simulink subsystem "s0307_theta_controller_PID"  (R2019b)
settings: Solver=VariableStepAuto  StartTime=0.0  StopTime=10.0  RelTol=1e-3
model mask{wc=0, cz_ratio=0, pc_ratio=0}
  mask prompts: wc "Cutting Frequency"; cz_ratio "Cutting/Zeros Frequency Ratio"; pc_ratio "Pole/Cutting Frequency Ratio"
undefined symbols (not defined in the file): dt_control, PARAMS
libraries: simulink x1
settings Model: Creator=paolo  LastModifiedBy=paolo
settings DebuggingCC: SFMachineParentedDataDiag=error

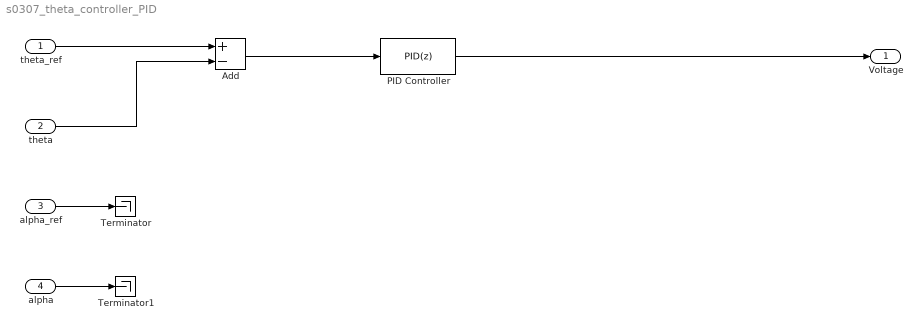
== system s0307_theta_controller_PID ==
  theta_ref : Inport
  theta : Inport  Port=2
  alpha_ref : Inport  Port=3
  alpha : Inport  Port=4
  Add : Sum  Inputs=+-
  PID Controller : simulink/Continuous/PID Controller  Controller=PID  Form=Parallel  TimeDomain=Discrete-time  SampleTime=dt_control  IntegratorMethod=Trapezoidal  FilterMethod=Trapezoidal  ControllerParametersSource=internal  P=wc^2 * (2 * cz_ratio * pc_ratio - 1) / (cz_ratio^2 * pc_ratio * PARAMS.mu_V_theta_dot)  I=wc^3 / PARAMS.mu_V_theta_dot / cz_ratio^2  D="wc * (cz_ratio^2 * pc_ratio^2 - 2 * cz_ratio * pc_ratio + 1)  / (cz_ratio^2 * pc_ratio^2 * PARAMS.mu_V_theta_dot)"  UseFilter=on  N=pc_ratio * wc  TunerSelectOption=Frequency Response Based  InitialConditionSource=internal  InitialConditionForIntegrator=0  InitialConditionForFilter=0  DifferentiatorICPrevScaledInput=0  ExternalReset=none  TrackingMode=off  Kt=1  LimitOutput=on  UpperSaturationLimit=PARAMS.V_sat  LowerSaturationLimit=-PARAMS.V_sat  LinearizeAsGain=on  AntiWindupMode=clamping  Kb=1  POutMin=[]  POutMax=[]  IOutMin=[]  IOutMax=[]  DOutMin=[]  DOutMax=[]  NOutMin=[]  NOutMax=[]  SumOutMin=[]  SumOutMax=[]  SaturationOutMin=[]  SaturationOutMax=[]  PParamMin=[]  PParamMax=[]  IParamMin=[]  IParamMax=[]  DParamMin=[]  DParamMax=[]  NParamMin=[]  NParamMax=[]  KbParamMin=[]  KbParamMax=[]  KtParamMin=[]  KtParamMax=[]  KbOutMin=[]  KbOutMax=[]  KtOutMin=[]  KtOutMax=[]  IntegratorOutMin=[]  IntegratorOutMax=[]  FilterOutMin=[]  FilterOutMax=[]  SumI1OutMin=[]  SumI1OutMax=[]  SumI2OutMin=[]  SumI2OutMax=[]  SumI3OutMin=[]  SumI3OutMax=[]  SumI4OutMin=[]  SumI4OutMax=[]  SumDOutMin=[]  SumDOutMax=[]  DifferentiatorOutMin=[]  DifferentiatorOutMax=[]  FilterDiffOutCoefMin=[]  FilterDiffOutCoefMax=[]  ReciprocalOutMin=[]  ReciprocalOutMax=[]  SumDenOutMin=[]  SumDenOutMax=[]  SumNumOutMin=[]  SumNumOutMax=[]  DivideOutMin=[]  DivideOutMax=[]  IntegratorContinuousStateAttributes=''  IntegratorStateMustResolveToSignalObject=off  IntegratorRTWStateStorageClass=Auto  FilterContinuousStateAttributes=''  FilterStateMustResolveToSignalObject=off  FilterRTWStateStorageClass=Auto  ParallelPVariant=InternalParameters  IdealPVariant=Disabled  IVariant=InternalParameters  DVariant=InternalParameters  IntegratorVariant=Discrete  SatVariant=Enabled  AWVariant=DiscClampingParallel  PCopyVariant=Disabled  TRVariant=Disabled  FdbkBlocksVariant=Feedback  IdealPFdbkVariant=Passthrough  SatFdbkVariant=Passthrough  DerivativeFilterVariant=TrapezoidalFilter  NVariant=InternalParameters  NCopyVariant=InternalParameters  FilterICVariant=InternalICsFilter  IntegratorICVariant=InternalICs  ExternalResetVariant=Disabled  TRSumVariant=Passthrough  SumFdbkVariant=Enabled  SumVariant=Sum_PID
  Terminator : Terminator
  Terminator1 : Terminator
  Voltage : Outport
  wires:
  Add/1 -> PID Controller/1
  theta/1 -> Add/2
  alpha_ref/1 -> Terminator/1
  alpha/1 -> Terminator1/1
  theta_ref/1 -> Add/1
  PID Controller/1 -> Voltage/1
